simulink model "CCH_PID_UNTUNED_outer"  (R2023a)
settings: Solver=VariableStepAuto  StartTime=0.0  StopTime=10.0  RelTol=1e-3
values from neighbouring files (symbols this model uses):
  AA = tlr{1}    [initLinCCH6dof.m]    (also in initalizeLinearCCH.m)
  BB = tlr{2}    [initLinCCH6dof.m]    (also in initalizeLinearCCH.m)
  CC = tlr{3}    [initLinCCH6dof.m]    (also in initalizeLinearCCH.m)
  DD = tlr{4}    [initLinCCH6dof.m]    (also in initalizeLinearCCH.m)
  epsilon = 0.0000001    (= 1e-07)    [coaxial_heli_parameters.m]    (also in nonLinearSimulation.m = 0.001)
  L_theta_c = TrimLinSave_6dof{idx_speed,2}(4,4)    [EMFController6dofSimulationBobAccelDecell.m]    (also in initLinCCH6dof.m = BB(4,4); nonLimSimFunction.m)
  M_delta_e = TrimLinSave{idx_speed,2}(3,4)    [EMFController3dofSimulation3211.m]    (also in EMFController6dofSimulationBobAccelDecell.m = TrimLinSave_6dof{idx_speed,2}(5,7); initLinCCH6dof.m = BB(5,7); initalizeLinearCCH.m = BB(3,4); nonLimSimFunction.m = TrimLinSave_6dof{idx_speed,2}(5,7))
  M_theta_s = TrimLinSave_6dof{idx_speed,2}(5,3)    [EMFController6dofSimulationBobAccelDecell.m]    (also in initLinCCH6dof.m = BB(5,3); initalizeLinearCCH.m = BB(3,2); nonLimSimFunction.m)
  N_delta_r = TrimLinSave_6dof{idx_speed,2}(6,8)    [EMFController6dofSimulationBobAccelDecell.m]    (also in initLinCCH6dof.m = BB(6,8); nonLimSimFunction.m)
  N_theta_d = TrimLinSave_6dof{idx_speed,2}(6,2)    [EMFController6dofSimulationBobAccelDecell.m]    (also in initLinCCH6dof.m = BB(6,2); nonLimSimFunction.m)
  V_l_transit = V_transit_save(1)    [EMFController3dofSimulation3211.m]    (also in EMFController6dofSimulationBobAccelDecell.m = V_transit_save(1)/1.94384; initLinCCH6dof.m; initalizeLinearCCH.m; nonLimSimFunction.m)
  V_u_transit = V_transit_save(2)-20    [EMFController3dofSimulation3211.m]    (also in EMFController6dofSimulationBobAccelDecell.m = V_transit_save(2)/1.94384-20; initLinCCH6dof.m = V_transit_save(2); initalizeLinearCCH.m = V_transit_save(2); nonLimSimFunction.m)
  X_theta_p = TrimLinSave{idx_speed,2}(1,3)    [EMFController3dofSimulation3211.m]    (also in EMFController6dofSimulationBobAccelDecell.m = TrimLinSave_6dof{idx_speed,2}(1,6); initLinCCH6dof.m = BB(1,6); nonLimSimFunction.m = TrimLinSave_6dof{idx_speed,2}(1,6))
  ytrim = ytrim(:,ii)    [initLinCCH6dof.m]
  Z_theta_0 = TrimLinSave{idx_speed,2}(2,1)    [EMFController3dofSimulation3211.m]    (also in EMFController6dofSimulationBobAccelDecell.m = TrimLinSave_6dof{idx_speed,2}(3,1); initLinCCH6dof.m = BB(3,1); nonLimSimFunction.m = TrimLinSave_6dof{idx_speed,2}(3,1))
libraries: slpidlib x9, SignalEditorBlockLib x2, simulink_extras x2
settings Model: Creator=prenc  LastModifiedBy=prenc

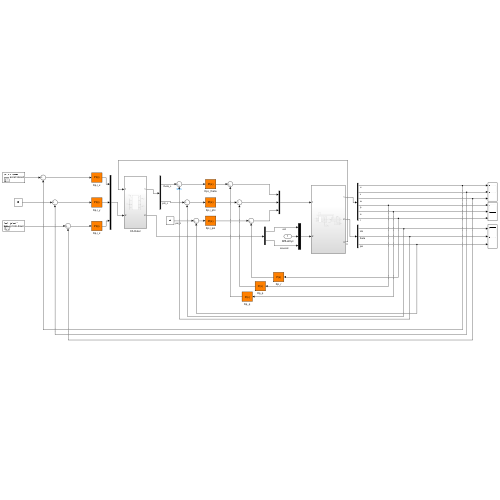
[thumbnail: Simulink's stored preview of the top-level diagram]
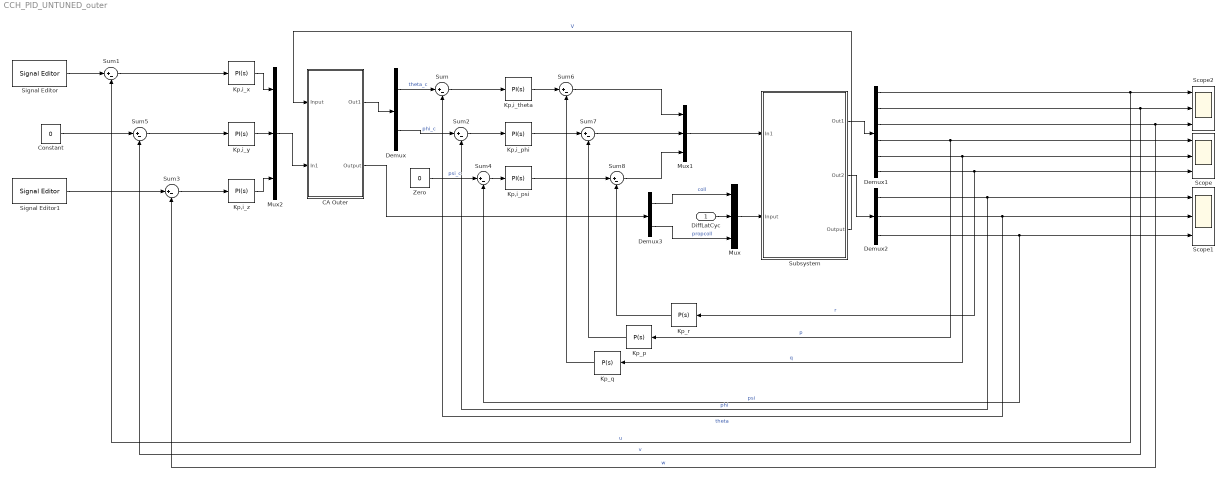
== system CCH_PID_UNTUNED_outer ==
  DiffLatCyc : Inport
  CA Outer : Subsystem
  Constant : Constant  Value=0
  Demux : Demux  Outputs=2
  Demux1 : Demux  Outputs=6
  Demux2 : Demux  Outputs=3
  Demux3 : Demux  Outputs=2
  Kp,i_phi : slpidlib/PID Controller  Controller=PI  Form=Parallel  TimeDomain=Continuous-time  UseExternalTs=off  SampleTime=-1  IntegratorMethod=Forward Euler  FilterMethod=Forward Euler  ControllerParametersSource=internal  P=0.271919090229755  I=18.9432812283601  UseKiTs=off  D=0  N=100  UseFilter=on  TunerSelectOption=Transfer Function Based (PID Tuner App)  InitialConditionSource=internal  InitialConditionForIntegrator=0  InitialConditionForFilter=0  DifferentiatorICPrevScaledInput=0  ExternalReset=none  TrackingMode=off  Kt=1  LimitOutput=off  SatLimitsSource=internal  UpperSaturationLimit=inf  LowerSaturationLimit=-inf  LinearizeAsGain=on  AntiWindupMode=none  Kb=1  LimitIntegrator=off  UpperIntegratorSaturationLimit=inf  LowerIntegratorSaturationLimit=-inf  POutMin=[]  POutMax=[]  IOutMin=[]  IOutMax=[]  DOutMin=[]  DOutMax=[]  NOutMin=[]  NOutMax=[]  SumOutMin=[]  SumOutMax=[]  SaturationOutMin=[]  SaturationOutMax=[]  PParamMin=[]  PParamMax=[]  IParamMin=[]  IParamMax=[]  DParamMin=[]  DParamMax=[]  NParamMin=[]  NParamMax=[]  KbParamMin=[]  KbParamMax=[]  KtParamMin=[]  KtParamMax=[]  KbOutMin=[]  KbOutMax=[]  KtOutMin=[]  KtOutMax=[]  IntegratorOutMin=[]  IntegratorOutMax=[]  FilterOutMin=[]  FilterOutMax=[]  SumI1OutMin=[]  SumI1OutMax=[]  SumI2OutMin=[]  SumI2OutMax=[]  SumI3OutMin=[]  SumI3OutMax=[]  SumI4OutMin=[]  SumI4OutMax=[]  SumDOutMin=[]  SumDOutMax=[]  DifferentiatorOutMin=[]  DifferentiatorOutMax=[]  FilterDiffOutCoefMin=[]  FilterDiffOutCoefMax=[]  ReciprocalOutMin=[]  ReciprocalOutMax=[]  SumDenOutMin=[]  SumDenOutMax=[]  SumNumOutMin=[]  SumNumOutMax=[]  DivideOutMin=[]  DivideOutMax=[]  UdiffTsProdOutMin=[]  UdiffTsProdOutMax=[]  NTsProdOutMin=[]  NTsProdOutMax=[]  UintegralTsProdOutMin=[]  UintegralTsProdOutMax=[]  UngainTsProdOutMin=[]  UngainTsProdOutMax=[]  ClampingZeroOutDataTypeStr=Inherit: Inherit via back propagation  ClampingZeroOutMin=[]  ClampingZeroOutMax=[]  FilterDenConstantOutDataTypeStr=Inherit: Inherit via back propagation  FilterDenConstantOutMin=[]  FilterDenConstantOutMax=[]  PCopyOutDataTypeStr=Inherit: Inherit via back propagation  PCopyOutMin=[]  PCopyOutMax=[]  NCopyOutDataTypeStr=Inherit: Inherit via back propagation  NCopyOutMin=[]  NCopyOutMax=[]  IntegratorContinuousStateAttributes=''  IntegratorStateMustResolveToSignalObject=off  IntegratorRTWStateStorageClass=Auto  FilterContinuousStateAttributes=''  FilterStateMustResolveToSignalObject=off  FilterRTWStateStorageClass=Auto  ParallelPVariant=InternalParameters  IdealPVariant=Disabled  IVariant=InternalParameters  DVariant=Disabled  IntegratorVariant=Continuous  SatVariant=Disabled  AWVariant=Passthrough  PCopyVariant=Disabled  TRVariant=Disabled  FdbkBlocksVariant=Forward  IdealPFdbkVariant=Disabled  SatFdbkVariant=Disabled  DerivativeFilterVariant=Disabled  NVariant=Disabled  NCopyVariant=Disabled_SignalSpec  FilterICVariant=Disabled  IntegratorICVariant=InternalICs  ExternalResetVariant=Disabled  TRSumVariant=Passthrough  SumFdbkVariant=Disabled  SumVariant=Sum_PI  TsampFilterVariant=InternalTs  TsampNgainVariant=Passthrough  TsampIntegralVariant=Disabled_SignalSpec  ExternalSaturationOutDataTypeStr=Inherit: Same as second input
  Kp,i_psi : slpidlib/PID Controller  Controller=PI  Form=Parallel  TimeDomain=Continuous-time  UseExternalTs=off  SampleTime=-1  IntegratorMethod=Forward Euler  FilterMethod=Forward Euler  ControllerParametersSource=internal  P=0.0996155787576819  I=3.12041407560122e-08  UseKiTs=off  D=0  N=100  UseFilter=on  TunerSelectOption=Transfer Function Based (PID Tuner App)  InitialConditionSource=internal  InitialConditionForIntegrator=0  InitialConditionForFilter=0  DifferentiatorICPrevScaledInput=0  ExternalReset=none  TrackingMode=off  Kt=1  LimitOutput=off  SatLimitsSource=internal  UpperSaturationLimit=inf  LowerSaturationLimit=-inf  LinearizeAsGain=on  AntiWindupMode=none  Kb=1  LimitIntegrator=off  UpperIntegratorSaturationLimit=inf  LowerIntegratorSaturationLimit=-inf  POutMin=[]  POutMax=[]  IOutMin=[]  IOutMax=[]  DOutMin=[]  DOutMax=[]  NOutMin=[]  NOutMax=[]  SumOutMin=[]  SumOutMax=[]  SaturationOutMin=[]  SaturationOutMax=[]  PParamMin=[]  PParamMax=[]  IParamMin=[]  IParamMax=[]  DParamMin=[]  DParamMax=[]  NParamMin=[]  NParamMax=[]  KbParamMin=[]  KbParamMax=[]  KtParamMin=[]  KtParamMax=[]  KbOutMin=[]  KbOutMax=[]  KtOutMin=[]  KtOutMax=[]  IntegratorOutMin=[]  IntegratorOutMax=[]  FilterOutMin=[]  FilterOutMax=[]  SumI1OutMin=[]  SumI1OutMax=[]  SumI2OutMin=[]  SumI2OutMax=[]  SumI3OutMin=[]  SumI3OutMax=[]  SumI4OutMin=[]  SumI4OutMax=[]  SumDOutMin=[]  SumDOutMax=[]  DifferentiatorOutMin=[]  DifferentiatorOutMax=[]  FilterDiffOutCoefMin=[]  FilterDiffOutCoefMax=[]  ReciprocalOutMin=[]  ReciprocalOutMax=[]  SumDenOutMin=[]  SumDenOutMax=[]  SumNumOutMin=[]  SumNumOutMax=[]  DivideOutMin=[]  DivideOutMax=[]  UdiffTsProdOutMin=[]  UdiffTsProdOutMax=[]  NTsProdOutMin=[]  NTsProdOutMax=[]  UintegralTsProdOutMin=[]  UintegralTsProdOutMax=[]  UngainTsProdOutMin=[]  UngainTsProdOutMax=[]  ClampingZeroOutDataTypeStr=Inherit: Inherit via back propagation  ClampingZeroOutMin=[]  ClampingZeroOutMax=[]  FilterDenConstantOutDataTypeStr=Inherit: Inherit via back propagation  FilterDenConstantOutMin=[]  FilterDenConstantOutMax=[]  PCopyOutDataTypeStr=Inherit: Inherit via back propagation  PCopyOutMin=[]  PCopyOutMax=[]  NCopyOutDataTypeStr=Inherit: Inherit via back propagation  NCopyOutMin=[]  NCopyOutMax=[]  IntegratorContinuousStateAttributes=''  IntegratorStateMustResolveToSignalObject=off  IntegratorRTWStateStorageClass=Auto  FilterContinuousStateAttributes=''  FilterStateMustResolveToSignalObject=off  FilterRTWStateStorageClass=Auto  ParallelPVariant=InternalParameters  IdealPVariant=Disabled  IVariant=InternalParameters  DVariant=Disabled  IntegratorVariant=Continuous  SatVariant=Disabled  AWVariant=Passthrough  PCopyVariant=Disabled  TRVariant=Disabled  FdbkBlocksVariant=Forward  IdealPFdbkVariant=Disabled  SatFdbkVariant=Disabled  DerivativeFilterVariant=Disabled  NVariant=Disabled  NCopyVariant=Disabled_SignalSpec  FilterICVariant=Disabled  IntegratorICVariant=InternalICs  ExternalResetVariant=Disabled  TRSumVariant=Passthrough  SumFdbkVariant=Disabled  SumVariant=Sum_PI  TsampFilterVariant=InternalTs  TsampNgainVariant=Passthrough  TsampIntegralVariant=Disabled_SignalSpec  ExternalSaturationOutDataTypeStr=Inherit: Same as second input
  Kp,i_theta : slpidlib/PID Controller  Controller=PI  Form=Parallel  TimeDomain=Continuous-time  UseExternalTs=off  SampleTime=-1  IntegratorMethod=Forward Euler  FilterMethod=Forward Euler  ControllerParametersSource=internal  P=12638.4701492349  I=0.0101786581860016  UseKiTs=off  D=0  N=100  UseFilter=on  TunerSelectOption=Transfer Function Based (PID Tuner App)  InitialConditionSource=internal  InitialConditionForIntegrator=0  InitialConditionForFilter=0  DifferentiatorICPrevScaledInput=0  ExternalReset=none  TrackingMode=off  Kt=1  LimitOutput=off  SatLimitsSource=internal  UpperSaturationLimit=inf  LowerSaturationLimit=-inf  LinearizeAsGain=on  AntiWindupMode=none  Kb=1  LimitIntegrator=off  UpperIntegratorSaturationLimit=inf  LowerIntegratorSaturationLimit=-inf  POutMin=[]  POutMax=[]  IOutMin=[]  IOutMax=[]  DOutMin=[]  DOutMax=[]  NOutMin=[]  NOutMax=[]  SumOutMin=[]  SumOutMax=[]  SaturationOutMin=[]  SaturationOutMax=[]  PParamMin=[]  PParamMax=[]  IParamMin=[]  IParamMax=[]  DParamMin=[]  DParamMax=[]  NParamMin=[]  NParamMax=[]  KbParamMin=[]  KbParamMax=[]  KtParamMin=[]  KtParamMax=[]  KbOutMin=[]  KbOutMax=[]  KtOutMin=[]  KtOutMax=[]  IntegratorOutMin=[]  IntegratorOutMax=[]  FilterOutMin=[]  FilterOutMax=[]  SumI1OutMin=[]  SumI1OutMax=[]  SumI2OutMin=[]  SumI2OutMax=[]  SumI3OutMin=[]  SumI3OutMax=[]  SumI4OutMin=[]  SumI4OutMax=[]  SumDOutMin=[]  SumDOutMax=[]  DifferentiatorOutMin=[]  DifferentiatorOutMax=[]  FilterDiffOutCoefMin=[]  FilterDiffOutCoefMax=[]  ReciprocalOutMin=[]  ReciprocalOutMax=[]  SumDenOutMin=[]  SumDenOutMax=[]  SumNumOutMin=[]  SumNumOutMax=[]  DivideOutMin=[]  DivideOutMax=[]  UdiffTsProdOutMin=[]  UdiffTsProdOutMax=[]  NTsProdOutMin=[]  NTsProdOutMax=[]  UintegralTsProdOutMin=[]  UintegralTsProdOutMax=[]  UngainTsProdOutMin=[]  UngainTsProdOutMax=[]  ClampingZeroOutDataTypeStr=Inherit: Inherit via back propagation  ClampingZeroOutMin=[]  ClampingZeroOutMax=[]  FilterDenConstantOutDataTypeStr=Inherit: Inherit via back propagation  FilterDenConstantOutMin=[]  FilterDenConstantOutMax=[]  PCopyOutDataTypeStr=Inherit: Inherit via back propagation  PCopyOutMin=[]  PCopyOutMax=[]  NCopyOutDataTypeStr=Inherit: Inherit via back propagation  NCopyOutMin=[]  NCopyOutMax=[]  IntegratorContinuousStateAttributes=''  IntegratorStateMustResolveToSignalObject=off  IntegratorRTWStateStorageClass=Auto  FilterContinuousStateAttributes=''  FilterStateMustResolveToSignalObject=off  FilterRTWStateStorageClass=Auto  ParallelPVariant=InternalParameters  IdealPVariant=Disabled  IVariant=InternalParameters  DVariant=Disabled  IntegratorVariant=Continuous  SatVariant=Disabled  AWVariant=Passthrough  PCopyVariant=Disabled  TRVariant=Disabled  FdbkBlocksVariant=Forward  IdealPFdbkVariant=Disabled  SatFdbkVariant=Disabled  DerivativeFilterVariant=Disabled  NVariant=Disabled  NCopyVariant=Disabled_SignalSpec  FilterICVariant=Disabled  IntegratorICVariant=InternalICs  ExternalResetVariant=Disabled  TRSumVariant=Passthrough  SumFdbkVariant=Disabled  SumVariant=Sum_PI  TsampFilterVariant=InternalTs  TsampNgainVariant=Passthrough  TsampIntegralVariant=Disabled_SignalSpec  ExternalSaturationOutDataTypeStr=Inherit: Same as second input
  Kp,i_x : slpidlib/PID Controller  Controller=PI  Form=Parallel  TimeDomain=Continuous-time  UseExternalTs=off  SampleTime=-1  IntegratorMethod=Forward Euler  FilterMethod=Forward Euler  ControllerParametersSource=internal  P=-0.593746516252291  I=-0.0342093441407178  UseKiTs=off  D=0  N=100  UseFilter=on  TunerSelectOption=Transfer Function Based (PID Tuner App)  InitialConditionSource=internal  InitialConditionForIntegrator=0  InitialConditionForFilter=0  DifferentiatorICPrevScaledInput=0  ExternalReset=none  TrackingMode=off  Kt=1  LimitOutput=off  SatLimitsSource=internal  UpperSaturationLimit=inf  LowerSaturationLimit=-inf  LinearizeAsGain=on  AntiWindupMode=none  Kb=1  LimitIntegrator=off  UpperIntegratorSaturationLimit=inf  LowerIntegratorSaturationLimit=-inf  POutMin=[]  POutMax=[]  IOutMin=[]  IOutMax=[]  DOutMin=[]  DOutMax=[]  NOutMin=[]  NOutMax=[]  SumOutMin=[]  SumOutMax=[]  SaturationOutMin=[]  SaturationOutMax=[]  PParamMin=[]  PParamMax=[]  IParamMin=[]  IParamMax=[]  DParamMin=[]  DParamMax=[]  NParamMin=[]  NParamMax=[]  KbParamMin=[]  KbParamMax=[]  KtParamMin=[]  KtParamMax=[]  KbOutMin=[]  KbOutMax=[]  KtOutMin=[]  KtOutMax=[]  IntegratorOutMin=[]  IntegratorOutMax=[]  FilterOutMin=[]  FilterOutMax=[]  SumI1OutMin=[]  SumI1OutMax=[]  SumI2OutMin=[]  SumI2OutMax=[]  SumI3OutMin=[]  SumI3OutMax=[]  SumI4OutMin=[]  SumI4OutMax=[]  SumDOutMin=[]  SumDOutMax=[]  DifferentiatorOutMin=[]  DifferentiatorOutMax=[]  FilterDiffOutCoefMin=[]  FilterDiffOutCoefMax=[]  ReciprocalOutMin=[]  ReciprocalOutMax=[]  SumDenOutMin=[]  SumDenOutMax=[]  SumNumOutMin=[]  SumNumOutMax=[]  DivideOutMin=[]  DivideOutMax=[]  UdiffTsProdOutMin=[]  UdiffTsProdOutMax=[]  NTsProdOutMin=[]  NTsProdOutMax=[]  UintegralTsProdOutMin=[]  UintegralTsProdOutMax=[]  UngainTsProdOutMin=[]  UngainTsProdOutMax=[]  ClampingZeroOutDataTypeStr=Inherit: Inherit via back propagation  ClampingZeroOutMin=[]  ClampingZeroOutMax=[]  FilterDenConstantOutDataTypeStr=Inherit: Inherit via back propagation  FilterDenConstantOutMin=[]  FilterDenConstantOutMax=[]  PCopyOutDataTypeStr=Inherit: Inherit via back propagation  PCopyOutMin=[]  PCopyOutMax=[]  NCopyOutDataTypeStr=Inherit: Inherit via back propagation  NCopyOutMin=[]  NCopyOutMax=[]  IntegratorContinuousStateAttributes=''  IntegratorStateMustResolveToSignalObject=off  IntegratorRTWStateStorageClass=Auto  FilterContinuousStateAttributes=''  FilterStateMustResolveToSignalObject=off  FilterRTWStateStorageClass=Auto  ParallelPVariant=InternalParameters  IdealPVariant=Disabled  IVariant=InternalParameters  DVariant=Disabled  IntegratorVariant=Continuous  SatVariant=Disabled  AWVariant=Passthrough  PCopyVariant=Disabled  TRVariant=Disabled  FdbkBlocksVariant=Forward  IdealPFdbkVariant=Disabled  SatFdbkVariant=Disabled  DerivativeFilterVariant=Disabled  NVariant=Disabled  NCopyVariant=Disabled_SignalSpec  FilterICVariant=Disabled  IntegratorICVariant=InternalICs  ExternalResetVariant=Disabled  TRSumVariant=Passthrough  SumFdbkVariant=Disabled  SumVariant=Sum_PI  TsampFilterVariant=InternalTs  TsampNgainVariant=Passthrough  TsampIntegralVariant=Disabled_SignalSpec  ExternalSaturationOutDataTypeStr=Inherit: Same as second input
  Kp,i_y : slpidlib/PID Controller  Controller=PI  Form=Parallel  TimeDomain=Continuous-time  UseExternalTs=off  SampleTime=-1  IntegratorMethod=Forward Euler  FilterMethod=Forward Euler  ControllerParametersSource=internal  P=7865.64876158662  I=-33.9330553860311  UseKiTs=off  D=0  N=100  UseFilter=on  TunerSelectOption=Transfer Function Based (PID Tuner App)  InitialConditionSource=internal  InitialConditionForIntegrator=0  InitialConditionForFilter=0  DifferentiatorICPrevScaledInput=0  ExternalReset=none  TrackingMode=off  Kt=1  LimitOutput=off  SatLimitsSource=internal  UpperSaturationLimit=inf  LowerSaturationLimit=-inf  LinearizeAsGain=on  AntiWindupMode=none  Kb=1  LimitIntegrator=off  UpperIntegratorSaturationLimit=inf  LowerIntegratorSaturationLimit=-inf  POutMin=[]  POutMax=[]  IOutMin=[]  IOutMax=[]  DOutMin=[]  DOutMax=[]  NOutMin=[]  NOutMax=[]  SumOutMin=[]  SumOutMax=[]  SaturationOutMin=[]  SaturationOutMax=[]  PParamMin=[]  PParamMax=[]  IParamMin=[]  IParamMax=[]  DParamMin=[]  DParamMax=[]  NParamMin=[]  NParamMax=[]  KbParamMin=[]  KbParamMax=[]  KtParamMin=[]  KtParamMax=[]  KbOutMin=[]  KbOutMax=[]  KtOutMin=[]  KtOutMax=[]  IntegratorOutMin=[]  IntegratorOutMax=[]  FilterOutMin=[]  FilterOutMax=[]  SumI1OutMin=[]  SumI1OutMax=[]  SumI2OutMin=[]  SumI2OutMax=[]  SumI3OutMin=[]  SumI3OutMax=[]  SumI4OutMin=[]  SumI4OutMax=[]  SumDOutMin=[]  SumDOutMax=[]  DifferentiatorOutMin=[]  DifferentiatorOutMax=[]  FilterDiffOutCoefMin=[]  FilterDiffOutCoefMax=[]  ReciprocalOutMin=[]  ReciprocalOutMax=[]  SumDenOutMin=[]  SumDenOutMax=[]  SumNumOutMin=[]  SumNumOutMax=[]  DivideOutMin=[]  DivideOutMax=[]  UdiffTsProdOutMin=[]  UdiffTsProdOutMax=[]  NTsProdOutMin=[]  NTsProdOutMax=[]  UintegralTsProdOutMin=[]  UintegralTsProdOutMax=[]  UngainTsProdOutMin=[]  UngainTsProdOutMax=[]  ClampingZeroOutDataTypeStr=Inherit: Inherit via back propagation  ClampingZeroOutMin=[]  ClampingZeroOutMax=[]  FilterDenConstantOutDataTypeStr=Inherit: Inherit via back propagation  FilterDenConstantOutMin=[]  FilterDenConstantOutMax=[]  PCopyOutDataTypeStr=Inherit: Inherit via back propagation  PCopyOutMin=[]  PCopyOutMax=[]  NCopyOutDataTypeStr=Inherit: Inherit via back propagation  NCopyOutMin=[]  NCopyOutMax=[]  IntegratorContinuousStateAttributes=''  IntegratorStateMustResolveToSignalObject=off  IntegratorRTWStateStorageClass=Auto  FilterContinuousStateAttributes=''  FilterStateMustResolveToSignalObject=off  FilterRTWStateStorageClass=Auto  ParallelPVariant=InternalParameters  IdealPVariant=Disabled  IVariant=InternalParameters  DVariant=Disabled  IntegratorVariant=Continuous  SatVariant=Disabled  AWVariant=Passthrough  PCopyVariant=Disabled  TRVariant=Disabled  FdbkBlocksVariant=Forward  IdealPFdbkVariant=Disabled  SatFdbkVariant=Disabled  DerivativeFilterVariant=Disabled  NVariant=Disabled  NCopyVariant=Disabled_SignalSpec  FilterICVariant=Disabled  IntegratorICVariant=InternalICs  ExternalResetVariant=Disabled  TRSumVariant=Passthrough  SumFdbkVariant=Disabled  SumVariant=Sum_PI  TsampFilterVariant=InternalTs  TsampNgainVariant=Passthrough  TsampIntegralVariant=Disabled_SignalSpec  ExternalSaturationOutDataTypeStr=Inherit: Same as second input
  Kp,i_z : slpidlib/PID Controller  Controller=PI  Form=Parallel  TimeDomain=Continuous-time  UseExternalTs=off  SampleTime=-1  IntegratorMethod=Forward Euler  FilterMethod=Forward Euler  ControllerParametersSource=internal  P=-0.271278935495006  I=-4.85135605851253e-09  UseKiTs=off  D=-1.00357554538256  N=68.8389227268809  UseFilter=on  TunerSelectOption=Transfer Function Based (PID Tuner App)  InitialConditionSource=internal  InitialConditionForIntegrator=0  InitialConditionForFilter=0  DifferentiatorICPrevScaledInput=0  ExternalReset=none  TrackingMode=off  Kt=1  LimitOutput=off  SatLimitsSource=internal  UpperSaturationLimit=inf  LowerSaturationLimit=-inf  LinearizeAsGain=on  AntiWindupMode=none  Kb=1  LimitIntegrator=off  UpperIntegratorSaturationLimit=inf  LowerIntegratorSaturationLimit=-inf  POutMin=[]  POutMax=[]  IOutMin=[]  IOutMax=[]  DOutMin=[]  DOutMax=[]  NOutMin=[]  NOutMax=[]  SumOutMin=[]  SumOutMax=[]  SaturationOutMin=[]  SaturationOutMax=[]  PParamMin=[]  PParamMax=[]  IParamMin=[]  IParamMax=[]  DParamMin=[]  DParamMax=[]  NParamMin=[]  NParamMax=[]  KbParamMin=[]  KbParamMax=[]  KtParamMin=[]  KtParamMax=[]  KbOutMin=[]  KbOutMax=[]  KtOutMin=[]  KtOutMax=[]  IntegratorOutMin=[]  IntegratorOutMax=[]  FilterOutMin=[]  FilterOutMax=[]  SumI1OutMin=[]  SumI1OutMax=[]  SumI2OutMin=[]  SumI2OutMax=[]  SumI3OutMin=[]  SumI3OutMax=[]  SumI4OutMin=[]  SumI4OutMax=[]  SumDOutMin=[]  SumDOutMax=[]  DifferentiatorOutMin=[]  DifferentiatorOutMax=[]  FilterDiffOutCoefMin=[]  FilterDiffOutCoefMax=[]  ReciprocalOutMin=[]  ReciprocalOutMax=[]  SumDenOutMin=[]  SumDenOutMax=[]  SumNumOutMin=[]  SumNumOutMax=[]  DivideOutMin=[]  DivideOutMax=[]  UdiffTsProdOutMin=[]  UdiffTsProdOutMax=[]  NTsProdOutMin=[]  NTsProdOutMax=[]  UintegralTsProdOutMin=[]  UintegralTsProdOutMax=[]  UngainTsProdOutMin=[]  UngainTsProdOutMax=[]  ClampingZeroOutDataTypeStr=Inherit: Inherit via back propagation  ClampingZeroOutMin=[]  ClampingZeroOutMax=[]  FilterDenConstantOutDataTypeStr=Inherit: Inherit via back propagation  FilterDenConstantOutMin=[]  FilterDenConstantOutMax=[]  PCopyOutDataTypeStr=Inherit: Inherit via back propagation  PCopyOutMin=[]  PCopyOutMax=[]  NCopyOutDataTypeStr=Inherit: Inherit via back propagation  NCopyOutMin=[]  NCopyOutMax=[]  IntegratorContinuousStateAttributes=''  IntegratorStateMustResolveToSignalObject=off  IntegratorRTWStateStorageClass=Auto  FilterContinuousStateAttributes=''  FilterStateMustResolveToSignalObject=off  FilterRTWStateStorageClass=Auto  ParallelPVariant=InternalParameters  IdealPVariant=Disabled  IVariant=InternalParameters  DVariant=Disabled  IntegratorVariant=Continuous  SatVariant=Disabled  AWVariant=Passthrough  PCopyVariant=Disabled  TRVariant=Disabled  FdbkBlocksVariant=Forward  IdealPFdbkVariant=Disabled  SatFdbkVariant=Disabled  DerivativeFilterVariant=Disabled  NVariant=Disabled  NCopyVariant=Disabled_SignalSpec  FilterICVariant=Disabled  IntegratorICVariant=InternalICs  ExternalResetVariant=Disabled  TRSumVariant=Passthrough  SumFdbkVariant=Disabled  SumVariant=Sum_PI  TsampFilterVariant=InternalTs  TsampNgainVariant=Passthrough  TsampIntegralVariant=Disabled_SignalSpec  ExternalSaturationOutDataTypeStr=Inherit: Same as second input
  Kp_p : slpidlib/PID Controller  Controller=P  Form=Parallel  TimeDomain=Continuous-time  UseExternalTs=off  SampleTime=-1  IntegratorMethod=Forward Euler  FilterMethod=Forward Euler  ControllerParametersSource=internal  P=73.2007341017675  I=-7.01634560053616e-07  UseKiTs=off  D=0  N=100  UseFilter=on  TunerSelectOption=Transfer Function Based (PID Tuner App)  InitialConditionSource=internal  InitialConditionForIntegrator=0  InitialConditionForFilter=0  DifferentiatorICPrevScaledInput=0  ExternalReset=none  TrackingMode=off  Kt=1  LimitOutput=off  SatLimitsSource=internal  UpperSaturationLimit=inf  LowerSaturationLimit=-inf  LinearizeAsGain=on  AntiWindupMode=none  Kb=1  LimitIntegrator=off  UpperIntegratorSaturationLimit=inf  LowerIntegratorSaturationLimit=-inf  POutMin=[]  POutMax=[]  IOutMin=[]  IOutMax=[]  DOutMin=[]  DOutMax=[]  NOutMin=[]  NOutMax=[]  SumOutMin=[]  SumOutMax=[]  SaturationOutMin=[]  SaturationOutMax=[]  PParamMin=[]  PParamMax=[]  IParamMin=[]  IParamMax=[]  DParamMin=[]  DParamMax=[]  NParamMin=[]  NParamMax=[]  KbParamMin=[]  KbParamMax=[]  KtParamMin=[]  KtParamMax=[]  KbOutMin=[]  KbOutMax=[]  KtOutMin=[]  KtOutMax=[]  IntegratorOutMin=[]  IntegratorOutMax=[]  FilterOutMin=[]  FilterOutMax=[]  SumI1OutMin=[]  SumI1OutMax=[]  SumI2OutMin=[]  SumI2OutMax=[]  SumI3OutMin=[]  SumI3OutMax=[]  SumI4OutMin=[]  SumI4OutMax=[]  SumDOutMin=[]  SumDOutMax=[]  DifferentiatorOutMin=[]  DifferentiatorOutMax=[]  FilterDiffOutCoefMin=[]  FilterDiffOutCoefMax=[]  ReciprocalOutMin=[]  ReciprocalOutMax=[]  SumDenOutMin=[]  SumDenOutMax=[]  SumNumOutMin=[]  SumNumOutMax=[]  DivideOutMin=[]  DivideOutMax=[]  UdiffTsProdOutMin=[]  UdiffTsProdOutMax=[]  NTsProdOutMin=[]  NTsProdOutMax=[]  UintegralTsProdOutMin=[]  UintegralTsProdOutMax=[]  UngainTsProdOutMin=[]  UngainTsProdOutMax=[]  ClampingZeroOutDataTypeStr=Inherit: Inherit via back propagation  ClampingZeroOutMin=[]  ClampingZeroOutMax=[]  FilterDenConstantOutDataTypeStr=Inherit: Inherit via back propagation  FilterDenConstantOutMin=[]  FilterDenConstantOutMax=[]  PCopyOutDataTypeStr=Inherit: Inherit via back propagation  PCopyOutMin=[]  PCopyOutMax=[]  NCopyOutDataTypeStr=Inherit: Inherit via back propagation  NCopyOutMin=[]  NCopyOutMax=[]  IntegratorContinuousStateAttributes=''  IntegratorStateMustResolveToSignalObject=off  IntegratorRTWStateStorageClass=Auto  FilterContinuousStateAttributes=''  FilterStateMustResolveToSignalObject=off  FilterRTWStateStorageClass=Auto  ParallelPVariant=InternalParameters  IdealPVariant=Disabled  IVariant=Disabled  DVariant=Disabled  IntegratorVariant=Disabled  SatVariant=Disabled  AWVariant=Disabled  PCopyVariant=Disabled  TRVariant=Disabled  FdbkBlocksVariant=Forward  IdealPFdbkVariant=Disabled  SatFdbkVariant=Disabled  DerivativeFilterVariant=Disabled  NVariant=Disabled  NCopyVariant=Disabled_SignalSpec  FilterICVariant=Disabled  IntegratorICVariant=Disabled  ExternalResetVariant=Disabled  TRSumVariant=Passthrough  SumFdbkVariant=Disabled  SumVariant=Passthrough_P  TsampFilterVariant=InternalTs  TsampNgainVariant=Passthrough  TsampIntegralVariant=Disabled_SignalSpec  ExternalSaturationOutDataTypeStr=Inherit: Same as second input
  Kp_q : slpidlib/PID Controller  Controller=P  Form=Parallel  TimeDomain=Continuous-time  UseExternalTs=off  SampleTime=-1  IntegratorMethod=Forward Euler  FilterMethod=Forward Euler  ControllerParametersSource=internal  P=174011.751166915  I=-7.01634560053616e-07  UseKiTs=off  D=0  N=100  UseFilter=on  TunerSelectOption=Transfer Function Based (PID Tuner App)  InitialConditionSource=internal  InitialConditionForIntegrator=0  InitialConditionForFilter=0  DifferentiatorICPrevScaledInput=0  ExternalReset=none  TrackingMode=off  Kt=1  LimitOutput=off  SatLimitsSource=internal  UpperSaturationLimit=inf  LowerSaturationLimit=-inf  LinearizeAsGain=on  AntiWindupMode=none  Kb=1  LimitIntegrator=off  UpperIntegratorSaturationLimit=inf  LowerIntegratorSaturationLimit=-inf  POutMin=[]  POutMax=[]  IOutMin=[]  IOutMax=[]  DOutMin=[]  DOutMax=[]  NOutMin=[]  NOutMax=[]  SumOutMin=[]  SumOutMax=[]  SaturationOutMin=[]  SaturationOutMax=[]  PParamMin=[]  PParamMax=[]  IParamMin=[]  IParamMax=[]  DParamMin=[]  DParamMax=[]  NParamMin=[]  NParamMax=[]  KbParamMin=[]  KbParamMax=[]  KtParamMin=[]  KtParamMax=[]  KbOutMin=[]  KbOutMax=[]  KtOutMin=[]  KtOutMax=[]  IntegratorOutMin=[]  IntegratorOutMax=[]  FilterOutMin=[]  FilterOutMax=[]  SumI1OutMin=[]  SumI1OutMax=[]  SumI2OutMin=[]  SumI2OutMax=[]  SumI3OutMin=[]  SumI3OutMax=[]  SumI4OutMin=[]  SumI4OutMax=[]  SumDOutMin=[]  SumDOutMax=[]  DifferentiatorOutMin=[]  DifferentiatorOutMax=[]  FilterDiffOutCoefMin=[]  FilterDiffOutCoefMax=[]  ReciprocalOutMin=[]  ReciprocalOutMax=[]  SumDenOutMin=[]  SumDenOutMax=[]  SumNumOutMin=[]  SumNumOutMax=[]  DivideOutMin=[]  DivideOutMax=[]  UdiffTsProdOutMin=[]  UdiffTsProdOutMax=[]  NTsProdOutMin=[]  NTsProdOutMax=[]  UintegralTsProdOutMin=[]  UintegralTsProdOutMax=[]  UngainTsProdOutMin=[]  UngainTsProdOutMax=[]  ClampingZeroOutDataTypeStr=Inherit: Inherit via back propagation  ClampingZeroOutMin=[]  ClampingZeroOutMax=[]  FilterDenConstantOutDataTypeStr=Inherit: Inherit via back propagation  FilterDenConstantOutMin=[]  FilterDenConstantOutMax=[]  PCopyOutDataTypeStr=Inherit: Inherit via back propagation  PCopyOutMin=[]  PCopyOutMax=[]  NCopyOutDataTypeStr=Inherit: Inherit via back propagation  NCopyOutMin=[]  NCopyOutMax=[]  IntegratorContinuousStateAttributes=''  IntegratorStateMustResolveToSignalObject=off  IntegratorRTWStateStorageClass=Auto  FilterContinuousStateAttributes=''  FilterStateMustResolveToSignalObject=off  FilterRTWStateStorageClass=Auto  ParallelPVariant=InternalParameters  IdealPVariant=Disabled  IVariant=Disabled  DVariant=Disabled  IntegratorVariant=Disabled  SatVariant=Disabled  AWVariant=Disabled  PCopyVariant=Disabled  TRVariant=Disabled  FdbkBlocksVariant=Forward  IdealPFdbkVariant=Disabled  SatFdbkVariant=Disabled  DerivativeFilterVariant=Disabled  NVariant=Disabled  NCopyVariant=Disabled_SignalSpec  FilterICVariant=Disabled  IntegratorICVariant=Disabled  ExternalResetVariant=Disabled  TRSumVariant=Passthrough  SumFdbkVariant=Disabled  SumVariant=Passthrough_P  TsampFilterVariant=InternalTs  TsampNgainVariant=Passthrough  TsampIntegralVariant=Disabled_SignalSpec  ExternalSaturationOutDataTypeStr=Inherit: Same as second input
  Kp_r : slpidlib/PID Controller  Controller=P  Form=Parallel  TimeDomain=Continuous-time  UseExternalTs=off  SampleTime=-1  IntegratorMethod=Forward Euler  FilterMethod=Forward Euler  ControllerParametersSource=internal  P=220.86619420845  I=-7.01634560053616e-07  UseKiTs=off  D=0  N=100  UseFilter=on  TunerSelectOption=Transfer Function Based (PID Tuner App)  InitialConditionSource=internal  InitialConditionForIntegrator=0  InitialConditionForFilter=0  DifferentiatorICPrevScaledInput=0  ExternalReset=none  TrackingMode=off  Kt=1  LimitOutput=off  SatLimitsSource=internal  UpperSaturationLimit=inf  LowerSaturationLimit=-inf  LinearizeAsGain=on  AntiWindupMode=none  Kb=1  LimitIntegrator=off  UpperIntegratorSaturationLimit=inf  LowerIntegratorSaturationLimit=-inf  POutMin=[]  POutMax=[]  IOutMin=[]  IOutMax=[]  DOutMin=[]  DOutMax=[]  NOutMin=[]  NOutMax=[]  SumOutMin=[]  SumOutMax=[]  SaturationOutMin=[]  SaturationOutMax=[]  PParamMin=[]  PParamMax=[]  IParamMin=[]  IParamMax=[]  DParamMin=[]  DParamMax=[]  NParamMin=[]  NParamMax=[]  KbParamMin=[]  KbParamMax=[]  KtParamMin=[]  KtParamMax=[]  KbOutMin=[]  KbOutMax=[]  KtOutMin=[]  KtOutMax=[]  IntegratorOutMin=[]  IntegratorOutMax=[]  FilterOutMin=[]  FilterOutMax=[]  SumI1OutMin=[]  SumI1OutMax=[]  SumI2OutMin=[]  SumI2OutMax=[]  SumI3OutMin=[]  SumI3OutMax=[]  SumI4OutMin=[]  SumI4OutMax=[]  SumDOutMin=[]  SumDOutMax=[]  DifferentiatorOutMin=[]  DifferentiatorOutMax=[]  FilterDiffOutCoefMin=[]  FilterDiffOutCoefMax=[]  ReciprocalOutMin=[]  ReciprocalOutMax=[]  SumDenOutMin=[]  SumDenOutMax=[]  SumNumOutMin=[]  SumNumOutMax=[]  DivideOutMin=[]  DivideOutMax=[]  UdiffTsProdOutMin=[]  UdiffTsProdOutMax=[]  NTsProdOutMin=[]  NTsProdOutMax=[]  UintegralTsProdOutMin=[]  UintegralTsProdOutMax=[]  UngainTsProdOutMin=[]  UngainTsProdOutMax=[]  ClampingZeroOutDataTypeStr=Inherit: Inherit via back propagation  ClampingZeroOutMin=[]  ClampingZeroOutMax=[]  FilterDenConstantOutDataTypeStr=Inherit: Inherit via back propagation  FilterDenConstantOutMin=[]  FilterDenConstantOutMax=[]  PCopyOutDataTypeStr=Inherit: Inherit via back propagation  PCopyOutMin=[]  PCopyOutMax=[]  NCopyOutDataTypeStr=Inherit: Inherit via back propagation  NCopyOutMin=[]  NCopyOutMax=[]  IntegratorContinuousStateAttributes=''  IntegratorStateMustResolveToSignalObject=off  IntegratorRTWStateStorageClass=Auto  FilterContinuousStateAttributes=''  FilterStateMustResolveToSignalObject=off  FilterRTWStateStorageClass=Auto  ParallelPVariant=InternalParameters  IdealPVariant=Disabled  IVariant=Disabled  DVariant=Disabled  IntegratorVariant=Disabled  SatVariant=Disabled  AWVariant=Disabled  PCopyVariant=Disabled  TRVariant=Disabled  FdbkBlocksVariant=Forward  IdealPFdbkVariant=Disabled  SatFdbkVariant=Disabled  DerivativeFilterVariant=Disabled  NVariant=Disabled  NCopyVariant=Disabled_SignalSpec  FilterICVariant=Disabled  IntegratorICVariant=Disabled  ExternalResetVariant=Disabled  TRSumVariant=Passthrough  SumFdbkVariant=Disabled  SumVariant=Passthrough_P  TsampFilterVariant=InternalTs  TsampNgainVariant=Passthrough  TsampIntegralVariant=Disabled_SignalSpec  ExternalSaturationOutDataTypeStr=Inherit: Same as second input
  Mux : Mux  Inputs=3
  Mux1 : Mux  Inputs=3
  Mux2 : Mux  Inputs=3
  Scope : Scope  NumInputPorts=3
  Scope1 : Scope  NumInputPorts=3
  Scope2 : Scope  NumInputPorts=3
  Signal Editor : SignalEditorBlockLib/Signal Editor  FileName=C:\Users\prenc\Documents\GitHub\CCHThesis\Generated Signals Simulink\bobupdown-acceldecell.mat  ActiveScenario=accellDecell  ActiveSignal=accell decell  IsBus=off  OutputBusObjectStr=Bus: BusObject  SampleTime=0  Interpolate=off  ZeroCross=off  OutputAfterFinalValue=Setting to zero  Unit=inherit  PreserveSignalName=on  ApplySigPropsToAllScenarios=on
  Signal Editor1 : SignalEditorBlockLib/Signal Editor  FileName=C:\Users\prenc\Documents\GitHub\CCHThesis\Generated Signals Simulink\bobupdown-acceldecell.mat  ActiveScenario=bobupdown  ActiveSignal=bob-up bob-down  IsBus=off  OutputBusObjectStr=Bus: BusObject  SampleTime=0  Interpolate=off  ZeroCross=off  OutputAfterFinalValue=Setting to zero  Unit=inherit  PreserveSignalName=on  ApplySigPropsToAllScenarios=on
  Subsystem : Subsystem
  Sum{,1..8} (9 alike) : Sum  Inputs=|+-
  Zero : Constant  Value=0  OutDataTypeStr=Inherit: Inherit via back propagation
  wires:
  Demux2/3 -> Scope1/3, Sum4/2  "psi"
  Kp_q/1 -> Sum6/2
  Kp_p/1 -> Sum7/2
  Kp,i_psi/1 -> Sum8/1
  Kp,i_phi/1 -> Sum7/1
  Demux3/1 -> Mux/1  "coll"
  DiffLatCyc/1 -> Mux/2
  Sum8/1 -> Mux1/3
  Demux1/2 -> Scope2/2, Sum5/2  "v"
  Demux2/2 -> Scope1/2, Sum/2  "theta"
  Demux3/2 -> Mux/3  "propcoll"
  Mux/1 -> Subsystem/2(Input)
  Sum7/1 -> Mux1/2
  Demux1/1 -> Scope2/1, Sum1/2  "u"
  Sum2/1 -> Kp,i_phi/1
  Subsystem/1(Out1) -> Demux1/1
  Sum6/1 -> Mux1/1
  Subsystem/2(Out2) -> Demux2/1
  Demux1/5 -> Scope/2, Kp_q/1  "q"
  Demux2/1 -> Scope1/1, Sum2/2  "phi"
  Kp_r/1 -> Sum8/2
  Sum/1 -> Kp,i_theta/1
  Sum4/1 -> Kp,i_psi/1
  Demux1/4 -> Scope/1, Kp_p/1  "p"
  Kp,i_theta/1 -> Sum6/1
  Demux/2 -> Sum2/1  "phi_c"
  Zero/1 -> Sum4/1  "psi_c"
  Demux1/6 -> Kp_r/1, Scope/3  "r"
  Mux1/1 -> Subsystem/1(In1)
  Demux/1 -> Sum/1  "theta_c"
  Demux1/3 -> Scope2/3, Sum3/2  "w"
  Signal Editor/1 -> Sum1/1
  Constant/1 -> Sum5/1
  Signal Editor1/1 -> Sum3/1
  Sum3/1 -> Kp,i_z/1
  Sum5/1 -> Kp,i_y/1
  Sum1/1 -> Kp,i_x/1
  Kp,i_z/1 -> Mux2/3
  Kp,i_y/1 -> Mux2/2
  Kp,i_x/1 -> Mux2/1
  CA Outer/1(Out1) -> Demux/1
  Mux2/1 -> CA Outer/2(In1)
  Subsystem/3(Output) -> CA Outer/1(Input)  "V"
  CA Outer/2(Output) -> Demux3/1

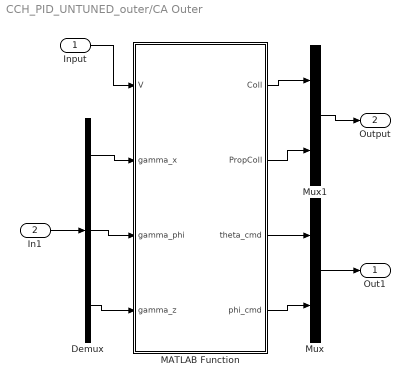
== system CCH_PID_UNTUNED_outer/CA Outer ==
  Input : Inport
  In1 : Inport  Port=2
  Demux : Demux  Outputs=3
  MATLAB Function : MATLAB Function  TreatAsAtomicUnit=on
  Mux : Mux  Inputs=2
  Mux1 : Mux  Inputs=2
  Out1 : Outport
  Output : Outport  Port=2
  wires:
  Input/1 -> MATLAB Function/1(V)
  In1/1 -> Demux/1
  Demux/1 -> MATLAB Function/2(gamma_x)
  Demux/2 -> MATLAB Function/3(gamma_phi)
  Demux/3 -> MATLAB Function/4(gamma_z)
  Mux/1 -> Out1/1
  MATLAB Function/2(PropColl) -> Mux1/2
  MATLAB Function/1(Coll) -> Mux1/1
  Mux1/1 -> Output/1
  MATLAB Function/3(theta_cmd) -> Mux/1
  MATLAB Function/4(phi_cmd) -> Mux/2

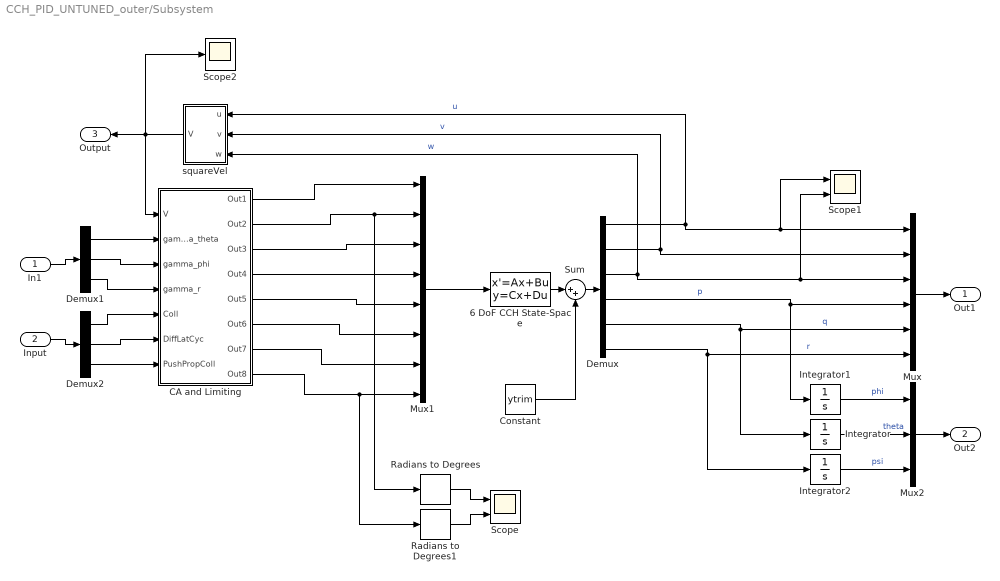
== system CCH_PID_UNTUNED_outer/Subsystem ==
  In1 : Inport
  Input : Inport  Port=2
  6 DoF CCH State-Space : StateSpace  A=AA  B=BB  C=CC  D=DD  InitialCondition=0
  CA and Limiting : Subsystem
  Constant : Constant  Value=ytrim
  Demux : Demux  Outputs=6
  Demux1 : Demux  Outputs=3
  Demux2 : Demux  Outputs=3
  Integrator : Integrator
  Integrator1 : Integrator
  Integrator2 : Integrator
  Mux : Mux  Inputs=6
  Mux1 : Mux  Inputs=8
  Mux2 : Mux  Inputs=3
  Radians to Degrees : simulink_extras/Transformations/Radians to Degrees
  Radians to Degrees1 : simulink_extras/Transformations/Radians to Degrees
  Scope : Scope  NumInputPorts=2
  Scope1 : Scope  NumInputPorts=2
  Scope2 : Scope
  Sum : Sum  Inputs=|++
  squareVel : MATLAB Function  TreatAsAtomicUnit=on
  Out1 : Outport
  Out2 : Outport  Port=2
  Output : Outport  Port=3
  wires:
  Mux/1 -> Out1/1
  CA and Limiting/7(Out7) -> Mux1/7
  Demux/5 -> Integrator/1, Mux/5  "q"
  CA and Limiting/2(Out2) -> Radians to Degrees/1, Mux1/2
  Demux/6 -> Mux/6, Integrator2/1  "r"
  Demux/3 -> squareVel/3(w), Scope1/2, Mux/3  "w"
  Demux/4 -> Integrator1/1, Mux/4  "p"
  CA and Limiting/1(Out1) -> Mux1/1
  Demux/2 -> squareVel/2(v), Mux/2  "v"
  Demux/1 -> squareVel/1(u), Scope1/1, Mux/1  "u"
  CA and Limiting/5(Out5) -> Mux1/5
  CA and Limiting/3(Out3) -> Mux1/3
  Mux1/1 -> 6 DoF CCH State-Space/1
  CA and Limiting/4(Out4) -> Mux1/4
  CA and Limiting/8(Out8) -> Radians to Degrees1/1, Mux1/8
  squareVel/1(V) -> Scope2/1, Output/1, CA and Limiting/1(V)
  CA and Limiting/6(Out6) -> Mux1/6
  Integrator2/1 -> Mux2/3  "psi"
  In1/1 -> Demux1/1
  Demux1/3 -> CA and Limiting/4(gamma_r)
  Demux1/1 -> CA and Limiting/2(gamma_theta)
  Demux1/2 -> CA and Limiting/3(gamma_phi)
  Demux2/1 -> CA and Limiting/5(Coll)
  Demux2/2 -> CA and Limiting/6(DiffLatCyc)
  Demux2/3 -> CA and Limiting/7(PushPropColl)
  Input/1 -> Demux2/1
  Mux2/1 -> Out2/1
  Integrator/1 -> Mux2/2  "theta"
  Integrator1/1 -> Mux2/1  "phi"
  Radians to Degrees/1 -> Scope/1
  Radians to Degrees1/1 -> Scope/2
  6 DoF CCH State-Space/1 -> Sum/1
  Sum/1 -> Demux/1
  Constant/1 -> Sum/2

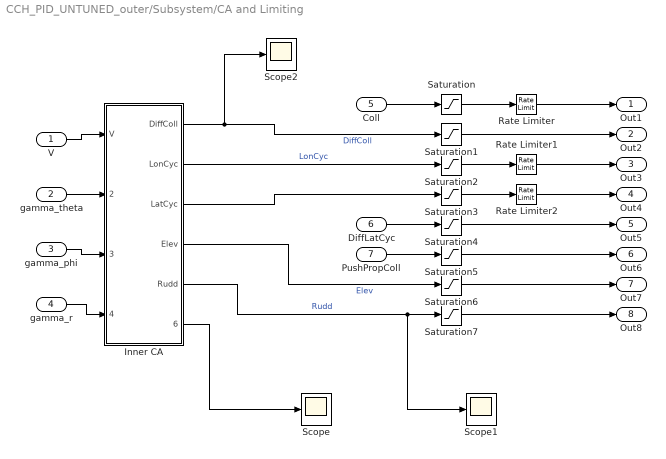
== system CCH_PID_UNTUNED_outer/Subsystem/CA and Limiting ==
  V : Inport
  gamma_theta : Inport  Port=2
  gamma_phi : Inport  Port=3
  gamma_r : Inport  Port=4
  Coll : Inport  Port=5
  DiffLatCyc : Inport  Port=6
  PushPropColl : Inport  Port=7
  Inner CA : MATLAB Function  TreatAsAtomicUnit=on
  Rate Limiter : RateLimiter  RisingSlewLimit=deg2rad(16)  FallingSlewLimit=deg2rad(-16)  SampleTimeMode=inherited
  Rate Limiter1 : RateLimiter  RisingSlewLimit=deg2rad(28.8)  FallingSlewLimit=deg2rad(-28.8)  SampleTimeMode=inherited
  Rate Limiter2 : RateLimiter  RisingSlewLimit=deg2rad(16)  FallingSlewLimit=deg2rad(-16)  SampleTimeMode=inherited
  Saturation : Saturate  UpperLimit=deg2rad(20)  LowerLimit=0
  Saturation1 : Saturate  UpperLimit=deg2rad(5)  LowerLimit=deg2rad(-5)
  Saturation2 : Saturate  UpperLimit=deg2rad(12)  LowerLimit=deg2rad(-12)
  Saturation3 : Saturate  UpperLimit=deg2rad(12)  LowerLimit=deg2rad(-12)
  Saturation4 : Saturate  UpperLimit=deg2rad(3)  LowerLimit=deg2rad(-3)
  Saturation5 : Saturate  UpperLimit=deg2rad(100)  LowerLimit=deg2rad(-10)
  Saturation6 : Saturate  UpperLimit=deg2rad(20)  LowerLimit=deg2rad(-20)
  Saturation7 : Saturate  UpperLimit=deg2rad(20)  LowerLimit=deg2rad(-20)
  Scope : Scope
  Scope1 : Scope
  Scope2 : Scope
  Out1 : Outport
  Out2 : Outport  Port=2
  Out3 : Outport  Port=3
  Out4 : Outport  Port=4
  Out5 : Outport  Port=5
  Out6 : Outport  Port=6
  Out7 : Outport  Port=7
  Out8 : Outport  Port=8
  wires:
  V/1 -> Inner CA/1(V)
  gamma_theta/1 -> Inner CA/2(gamma_theta)
  gamma_phi/1 -> Inner CA/3(gamma_phi)
  gamma_r/1 -> Inner CA/4(gamma_r)
  Rate Limiter1/1 -> Out3/1
  Saturation/1 -> Rate Limiter/1
  Saturation6/1 -> Out7/1
  Saturation3/1 -> Rate Limiter2/1
  Saturation2/1 -> Rate Limiter1/1
  Saturation5/1 -> Out6/1
  Saturation4/1 -> Out5/1
  Saturation1/1 -> Out2/1
  Inner CA/5(Rudd) -> Scope1/1, Saturation7/1  "Rudd"
  Inner CA/2(LonCyc) -> Saturation2/1  "LonCyc"
  DiffLatCyc/1 -> Saturation4/1
  Coll/1 -> Saturation/1
  PushPropColl/1 -> Saturation5/1
  Inner CA/4(Elev) -> Saturation6/1  "Elev"
  Saturation7/1 -> Out8/1
  Inner CA/3(LatCyc) -> Saturation3/1
  Inner CA/1(DiffColl) -> Scope2/1, Saturation1/1  "DiffColl"
  Rate Limiter2/1 -> Out4/1
  Rate Limiter/1 -> Out1/1
  Inner CA/6(rho_theta_d) -> Scope/1

== matlab function CCH_PID_UNTUNED_outer/Subsystem/squareVel ==
  data: u input; V output; v input; w input; trimvelocity parameter
function V = fcn(u,v,w, trimvelocity)

V = sqrt(u^2+v^2+w^2);

== matlab function CCH_PID_UNTUNED_outer/Subsystem/CA and Limiting/Inner CA ==
  data: DiffColl output; V input; LonCyc output; LatCyc output; gamma_theta input; gamma_phi input; gamma_r input; Elev output; V_l_transit parameter; epsilon parameter; V_u_transit parameter; M_theta_s parameter; M_delta_e parameter; Rudd output; L_theta_c parameter; N_theta_d parameter; N_delta_r parameter; rho_theta_d output
function [DiffColl, LonCyc, LatCyc, Elev, Rudd, rho_theta_d] = fcn(V, gamma_theta, gamma_phi, gamma_r, V_l_transit, epsilon, V_u_transit, M_theta_s, M_delta_e, L_theta_c, N_theta_d, N_delta_r)
    
    % Allocation Weights
    if V<V_l_transit
        rho_theta_c = 1;
        rho_delta_e = epsilon;

        rho_theta_d = 1;
        rho_delta_r = epsilon;

    elseif V>V_l_transit && V<V_u_transit
        rho_theta_c = 1 - 1/(V_u_transit-V_l_transit)*(V-V_l_transit);
        rho_delta_e = 1/(V_u_transit-V_l_transit)*(V-V_l_transit);

        rho_theta_d = 1 - 1/(V_u_transit-V_l_transit)*(V-V_l_transit);
        rho_delta_r = 1/(V_u_transit-V_l_transit)*(V-V_l_transit);
    else
        rho_theta_c = epsilon;
        rho_delta_e = 1;

        rho_theta_d = epsilon;
        rho_delta_r = 1;
    end

    % Pitch
    B_theta = [M_theta_s, M_delta_e];
    W_theta = [1/rho_theta_c, 0; 0, 1/rho_delta_e];
    U_theta = inv(W_theta)*transpose(B_theta)*inv(B_theta*inv(W_theta)*transpose(B_theta))*gamma_theta;

    LonCyc = U_theta(1);
    Elev = U_theta(2); 

    % Roll
    LatCyc = gamma_phi/L_theta_c;

    % Yaw
    B_psi = [N_theta_d, N_delta_r];
    W_psi = [1/rho_theta_d, 0; 0, 1/rho_delta_r];
    U_psi = inv(W_psi)*transpose(B_psi)* ...
        inv(B_psi*inv(W_psi)*transpose(B_psi))*gamma_r;
    DiffColl = U_psi(1);
    Rudd = U_psi(2);

== matlab function CCH_PID_UNTUNED_outer/CA Outer/MATLAB Function ==
  data: V input; Coll output; gamma_x input; gamma_phi input; gamma_z input; PropColl output; theta_cmd output; phi_cmd output; X_theta_p parameter; Z_theta_0 parameter; V_u_transit parameter; epsilon parameter; V_l_transit parameter; L_theta_c parameter
function [Coll, PropColl, theta_cmd, phi_cmd] = fcn(V, gamma_x, gamma_phi, gamma_z, X_theta_p, Z_theta_0, V_u_transit, epsilon, V_l_transit, L_theta_c)
    
    % Allocation Weights
    if V<V_l_transit
        rho_theta_x_cmd = 1;
        rho_theta_p = epsilon;

        rho_theta_0 = 1;
        rho_theta_z_cmd = epsilon;

    elseif V>V_l_transit && V<V_u_transit
        rho_theta_x_cmd = 1 - 1/(V_u_transit-V_l_transit)*(V-V_l_transit);
        rho_theta_p = 1/(V_u_transit-V_l_transit)*(V-V_l_transit);

        rho_theta_0 = 1 - 1/(V_u_transit-V_l_transit)*(V-V_l_transit);
        rho_theta_z_cmd = 1/(V_u_transit-V_l_transit)*(V-V_l_transit);
    else
        rho_theta_x_cmd = epsilon;
        rho_theta_p = 1;

        rho_theta_0 = epsilon;
        rho_theta_z_cmd = 1;
    end

    % LonVel
    B_x = [1, -X_theta_p];
    W_x = [1/rho_theta_x_cmd, 0; 0, 1/rho_theta_p];
    U_x = inv(W_x)*transpose(B_x)* inv(B_x*inv(W_x)*transpose(B_x))*gamma_x;

    theta_x_cmd = U_x(1);
    PropColl = U_x(2);

    % Height
    B_z = [Z_theta_0, 1];
    W_z = [1/rho_theta_0, 0; 0, 1/rho_theta_z_cmd];
    U_z = inv(W_z)*transpose(B_z)*inv(B_z*inv(W_z)*transpose(B_z))*gamma_z;
    
    Coll = U_z(1);
    theta_z_cmd = U_z(2);

    theta_cmd = theta_x_cmd+theta_z_cmd;

    % Roll
    phi_cmd = gamma_phi/L_theta_c;
